simulink model "Radar410_Rx"  (R2018b)
settings: Solver=VariableStepAuto  StartTime=0.0  StopTime=10.0  RelTol=1e-3
PostLoadFcn:
  | if any(exist('dsrtsu_mdlpostloadfcn', 'file') ~= 0), dsrtsu_mdlpostloadfcn('Execute', bdroot); end
libraries: rtican x82
(part 24 of 24)

== system Radar410_Rx/Radar410_RX/Subsystem41/Subsystem40 ==
  In1 : Inport
  Bus Creator : BusCreator  Inputs=11  OutDataTypeStr=Bus: Radar_Status  NonVirtualBus=on
      settings: InheritFromInputs=off
  Bus Selector : BusSelector  OutputSignals=FRS_Msg_CheckSum,FRS_Msg_AliveCounter,FRS_Status_MisAlign,FRS_Status_HWErr,FRS_Status_BlkProg,FRS_Fail,FRS_MeasEnabled,FRS_Host_Yaw,FRS_HostSpeed,FRS_TimeStamp,FRS_Latency
  Data Type Conversion{,1..10} (11 alike) : DataTypeConversion  OutDataTypeStr=single
  Out1 : Outport  OutDataTypeStr=Bus: Radar_Status
  wires:
  Bus Selector/5 -> Data Type Conversion4/1  "<FRS_Status_BlkProg>"
  Bus Selector/8 -> Data Type Conversion7/1  "<FRS_Host_Yaw>"
  Bus Selector/1 -> Data Type Conversion/1  "<FRS_Msg_CheckSum>"
  Bus Selector/3 -> Data Type Conversion2/1  "<FRS_Status_MisAlign>"
  Bus Selector/2 -> Data Type Conversion1/1  "<FRS_Msg_AliveCounter>"
  Data Type Conversion5/1 -> Bus Creator/6
  Bus Selector/4 -> Data Type Conversion3/1  "<FRS_Status_HWErr>"
  Bus Selector/7 -> Data Type Conversion6/1  "<FRS_MeasEnabled>"
  Data Type Conversion9/1 -> Bus Creator/10
  Bus Selector/6 -> Data Type Conversion5/1  "<FRS_Fail>"
  Bus Selector/11 -> Data Type Conversion10/1  "<FRS_Latency>"
  Data Type Conversion6/1 -> Bus Creator/7
  Bus Selector/9 -> Data Type Conversion8/1  "<FRS_HostSpeed>"
  Bus Selector/10 -> Data Type Conversion9/1  "<FRS_TimeStamp>"
  Data Type Conversion10/1 -> Bus Creator/11
  In1/1 -> Bus Selector/1
  Bus Creator/1 -> Out1/1
  Data Type Conversion/1 -> Bus Creator/1
  Data Type Conversion2/1 -> Bus Creator/3
  Data Type Conversion1/1 -> Bus Creator/2
  Data Type Conversion4/1 -> Bus Creator/5
  Data Type Conversion3/1 -> Bus Creator/4
  Data Type Conversion7/1 -> Bus Creator/8
  Data Type Conversion8/1 -> Bus Creator/9

== system Radar410_Rx/Radar410_RX/Subsystem41/Subsystem5 ==
  In1 : Inport
  Bus Creator : BusCreator  Inputs=20  OutDataTypeStr=Bus: Obj_Data  NonVirtualBus=on
      settings: InheritFromInputs=off
  Bus Selector : BusSelector  OutputSignals=FRS_P1_05_Msg_CheckSum,FRS_P1_05_Msg_AliveCounter,FRS_P1_05_Obj_ExstProb,FRS_P1_05_Obj_XVelRel_Stdev,FRS_P1_05_Obj_XAccRel,FRS_P1_05_Obj_ObstacleProb,FRS_P1_05_Obj_MotionPattern,FRS_P1_05_Obj_YPos_Stdev,FRS_P1_05_Obj_ValidFlag,FRS_P1_05_Obj_XPos_Stdev,FRS_P1_05_Obj_UpdateFlag,FRS_P1_05_Obj_ID,FRS_P2_05_Msg_CheckSum,FRS_P2_05_Msg_AliveCounter,FRS_P2_05_Obj_MeasFlag,FRS_P2_05_Obj_YVelRel,FRS_P2_05_Obj_Type,FRS_P2_05_Obj_XPos,FRS_P2_05_Obj_YPos,FRS_P2_05_Obj_XVelRel
  Data Type Conversion{,1..19} (20 alike) : DataTypeConversion  OutDataTypeStr=single
  Out1 : Outport  OutDataTypeStr=Bus: Obj_Data
  wires:
  Data Type Conversion19/1 -> Bus Creator/20
  Data Type Conversion14/1 -> Bus Creator/15
  Data Type Conversion8/1 -> Bus Creator/9
  Data Type Conversion7/1 -> Bus Creator/8
  Data Type Conversion3/1 -> Bus Creator/4
  Data Type Conversion4/1 -> Bus Creator/5
  Data Type Conversion1/1 -> Bus Creator/2
  Data Type Conversion13/1 -> Bus Creator/14
  Data Type Conversion2/1 -> Bus Creator/3
  Data Type Conversion/1 -> Bus Creator/1
  Bus Creator/1 -> Out1/1
  In1/1 -> Bus Selector/1
  Bus Selector/20 -> Data Type Conversion19/1  "<FRS_P2_05_Obj_XVelRel>"
  Bus Selector/18 -> Data Type Conversion17/1  "<FRS_P2_05_Obj_XPos>"
  Bus Selector/19 -> Data Type Conversion18/1  "<FRS_P2_05_Obj_YPos>"
  Bus Selector/14 -> Data Type Conversion13/1  "<FRS_P2_05_Msg_AliveCounter>"
  Data Type Conversion10/1 -> Bus Creator/11
  Bus Selector/10 -> Data Type Conversion9/1  "<FRS_P1_05_Obj_XPos_Stdev>"
  Bus Selector/17 -> Data Type Conversion16/1  "<FRS_P2_05_Obj_Type>"
  Bus Selector/9 -> Data Type Conversion8/1  "<FRS_P1_05_Obj_ValidFlag>"
  Data Type Conversion16/1 -> Bus Creator/17
  Bus Selector/12 -> Data Type Conversion11/1  "<FRS_P1_05_Obj_ID>"
  Data Type Conversion6/1 -> Bus Creator/7
  Bus Selector/16 -> Data Type Conversion15/1  "<FRS_P2_05_Obj_YVelRel>"
  Data Type Conversion17/1 -> Bus Creator/18
  Bus Selector/11 -> Data Type Conversion10/1  "<FRS_P1_05_Obj_UpdateFlag>"
  Data Type Conversion18/1 -> Bus Creator/19
  Bus Selector/6 -> Data Type Conversion5/1  "<FRS_P1_05_Obj_ObstacleProb>"
  Data Type Conversion9/1 -> Bus Creator/10
  Bus Selector/7 -> Data Type Conversion6/1  "<FRS_P1_05_Obj_MotionPattern>"
  Bus Selector/4 -> Data Type Conversion3/1  "<FRS_P1_05_Obj_XVelRel_Stdev>"
  Data Type Conversion5/1 -> Bus Creator/6
  Data Type Conversion11/1 -> Bus Creator/12
  Bus Selector/2 -> Data Type Conversion1/1  "<FRS_P1_05_Msg_AliveCounter>"
  Bus Selector/13 -> Data Type Conversion12/1  "<FRS_P2_05_Msg_CheckSum>"
  Bus Selector/3 -> Data Type Conversion2/1  "<FRS_P1_05_Obj_ExstProb>"
  Bus Selector/15 -> Data Type Conversion14/1  "<FRS_P2_05_Obj_MeasFlag>"
  Bus Selector/1 -> Data Type Conversion/1  "<FRS_P1_05_Msg_CheckSum>"
  Data Type Conversion15/1 -> Bus Creator/16
  Bus Selector/8 -> Data Type Conversion7/1  "<FRS_P1_05_Obj_YPos_Stdev>"
  Bus Selector/5 -> Data Type Conversion4/1  "<FRS_P1_05_Obj_XAccRel>"
  Data Type Conversion12/1 -> Bus Creator/13

== system Radar410_Rx/Radar410_RX/Subsystem41/Subsystem6 ==
  In1 : Inport
  Bus Creator : BusCreator  Inputs=20  OutDataTypeStr=Bus: Obj_Data  NonVirtualBus=on
      settings: InheritFromInputs=off
  Bus Selector : BusSelector  OutputSignals=FRS_P1_06_Msg_CheckSum,FRS_P1_06_Msg_AliveCounter,FRS_P1_06_Obj_ExstProb,FRS_P1_06_Obj_XVelRel_Stdev,FRS_P1_06_Obj_XAccRel,FRS_P1_06_Obj_ObstacleProb,FRS_P1_06_Obj_MotionPattern,FRS_P1_06_Obj_YPos_Stdev,FRS_P1_06_Obj_ValidFlag,FRS_P1_06_Obj_XPos_Stdev,FRS_P1_06_Obj_UpdateFlag,FRS_P1_06_Obj_ID,FRS_P2_06_Msg_CheckSum,FRS_P2_06_Msg_AliveCounter,FRS_P2_06_Obj_MeasFlag,FRS_P2_06_Obj_YVelRel,FRS_P2_06_Obj_Type,FRS_P2_06_Obj_XPos,FRS_P2_06_Obj_YPos,FRS_P2_06_Obj_XVelRel
  Data Type Conversion{,1..19} (20 alike) : DataTypeConversion  OutDataTypeStr=single
  Out1 : Outport  OutDataTypeStr=Bus: Obj_Data
  wires:
  Data Type Conversion19/1 -> Bus Creator/20
  Data Type Conversion14/1 -> Bus Creator/15
  Data Type Conversion8/1 -> Bus Creator/9
  Data Type Conversion7/1 -> Bus Creator/8
  Data Type Conversion3/1 -> Bus Creator/4
  Data Type Conversion4/1 -> Bus Creator/5
  Data Type Conversion1/1 -> Bus Creator/2
  Data Type Conversion13/1 -> Bus Creator/14
  Data Type Conversion2/1 -> Bus Creator/3
  Data Type Conversion/1 -> Bus Creator/1
  Bus Creator/1 -> Out1/1
  In1/1 -> Bus Selector/1
  Bus Selector/20 -> Data Type Conversion19/1  "<FRS_P2_06_Obj_XVelRel>"
  Bus Selector/18 -> Data Type Conversion17/1  "<FRS_P2_06_Obj_XPos>"
  Bus Selector/19 -> Data Type Conversion18/1  "<FRS_P2_06_Obj_YPos>"
  Bus Selector/14 -> Data Type Conversion13/1  "<FRS_P2_06_Msg_AliveCounter>"
  Data Type Conversion10/1 -> Bus Creator/11
  Bus Selector/10 -> Data Type Conversion9/1  "<FRS_P1_06_Obj_XPos_Stdev>"
  Bus Selector/17 -> Data Type Conversion16/1  "<FRS_P2_06_Obj_Type>"
  Bus Selector/9 -> Data Type Conversion8/1  "<FRS_P1_06_Obj_ValidFlag>"
  Data Type Conversion16/1 -> Bus Creator/17
  Bus Selector/12 -> Data Type Conversion11/1  "<FRS_P1_06_Obj_ID>"
  Data Type Conversion6/1 -> Bus Creator/7
  Bus Selector/16 -> Data Type Conversion15/1  "<FRS_P2_06_Obj_YVelRel>"
  Data Type Conversion17/1 -> Bus Creator/18
  Bus Selector/11 -> Data Type Conversion10/1  "<FRS_P1_06_Obj_UpdateFlag>"
  Data Type Conversion18/1 -> Bus Creator/19
  Bus Selector/6 -> Data Type Conversion5/1  "<FRS_P1_06_Obj_ObstacleProb>"
  Data Type Conversion9/1 -> Bus Creator/10
  Bus Selector/7 -> Data Type Conversion6/1  "<FRS_P1_06_Obj_MotionPattern>"
  Bus Selector/4 -> Data Type Conversion3/1  "<FRS_P1_06_Obj_XVelRel_Stdev>"
  Data Type Conversion5/1 -> Bus Creator/6
  Data Type Conversion11/1 -> Bus Creator/12
  Bus Selector/2 -> Data Type Conversion1/1  "<FRS_P1_06_Msg_AliveCounter>"
  Bus Selector/13 -> Data Type Conversion12/1  "<FRS_P2_06_Msg_CheckSum>"
  Bus Selector/3 -> Data Type Conversion2/1  "<FRS_P1_06_Obj_ExstProb>"
  Bus Selector/15 -> Data Type Conversion14/1  "<FRS_P2_06_Obj_MeasFlag>"
  Bus Selector/1 -> Data Type Conversion/1  "<FRS_P1_06_Msg_CheckSum>"
  Data Type Conversion15/1 -> Bus Creator/16
  Bus Selector/8 -> Data Type Conversion7/1  "<FRS_P1_06_Obj_YPos_Stdev>"
  Bus Selector/5 -> Data Type Conversion4/1  "<FRS_P1_06_Obj_XAccRel>"
  Data Type Conversion12/1 -> Bus Creator/13

== system Radar410_Rx/Radar410_RX/Subsystem41/Subsystem7 ==
  In1 : Inport
  Bus Creator : BusCreator  Inputs=20  OutDataTypeStr=Bus: Obj_Data  NonVirtualBus=on
      settings: InheritFromInputs=off
  Bus Selector : BusSelector  OutputSignals=FRS_P1_07_Msg_CheckSum,FRS_P1_07_Msg_AliveCounter,FRS_P1_07_Obj_ExstProb,FRS_P1_07_Obj_XVelRel_Stdev,FRS_P1_07_Obj_XAccRel,FRS_P1_07_Obj_ObstacleProb,FRS_P1_07_Obj_MotionPattern,FRS_P1_07_Obj_YPos_Stdev,FRS_P1_07_Obj_ValidFlag,FRS_P1_07_Obj_XPos_Stdev,FRS_P1_07_Obj_UpdateFlag,FRS_P1_07_Obj_ID,FRS_P2_07_Msg_CheckSum,FRS_P2_07_Msg_AliveCounter,FRS_P2_07_Obj_MeasFlag,FRS_P2_07_Obj_YVelRel,FRS_P2_07_Obj_Type,FRS_P2_07_Obj_XPos,FRS_P2_07_Obj_YPos,FRS_P2_07_Obj_XVelRel
  Data Type Conversion{,1..19} (20 alike) : DataTypeConversion  OutDataTypeStr=single
  Out1 : Outport  OutDataTypeStr=Bus: Obj_Data
  wires:
  Data Type Conversion12/1 -> Bus Creator/13
  Bus Selector/5 -> Data Type Conversion4/1  "<FRS_P1_07_Obj_XAccRel>"
  Bus Selector/8 -> Data Type Conversion7/1  "<FRS_P1_07_Obj_YPos_Stdev>"
  Data Type Conversion15/1 -> Bus Creator/16
  Bus Selector/1 -> Data Type Conversion/1  "<FRS_P1_07_Msg_CheckSum>"
  Bus Selector/15 -> Data Type Conversion14/1  "<FRS_P2_07_Obj_MeasFlag>"
  Bus Selector/3 -> Data Type Conversion2/1  "<FRS_P1_07_Obj_ExstProb>"
  Bus Selector/13 -> Data Type Conversion12/1  "<FRS_P2_07_Msg_CheckSum>"
  Bus Selector/2 -> Data Type Conversion1/1  "<FRS_P1_07_Msg_AliveCounter>"
  Data Type Conversion11/1 -> Bus Creator/12
  Data Type Conversion5/1 -> Bus Creator/6
  Bus Selector/4 -> Data Type Conversion3/1  "<FRS_P1_07_Obj_XVelRel_Stdev>"
  Bus Selector/7 -> Data Type Conversion6/1  "<FRS_P1_07_Obj_MotionPattern>"
  Data Type Conversion9/1 -> Bus Creator/10
  Bus Selector/6 -> Data Type Conversion5/1  "<FRS_P1_07_Obj_ObstacleProb>"
  Data Type Conversion18/1 -> Bus Creator/19
  Bus Selector/11 -> Data Type Conversion10/1  "<FRS_P1_07_Obj_UpdateFlag>"
  Data Type Conversion17/1 -> Bus Creator/18
  Bus Selector/16 -> Data Type Conversion15/1  "<FRS_P2_07_Obj_YVelRel>"
  Data Type Conversion6/1 -> Bus Creator/7
  Bus Selector/12 -> Data Type Conversion11/1  "<FRS_P1_07_Obj_ID>"
  Data Type Conversion16/1 -> Bus Creator/17
  Bus Selector/9 -> Data Type Conversion8/1  "<FRS_P1_07_Obj_ValidFlag>"
  Bus Selector/17 -> Data Type Conversion16/1  "<FRS_P2_07_Obj_Type>"
  Bus Selector/10 -> Data Type Conversion9/1  "<FRS_P1_07_Obj_XPos_Stdev>"
  Data Type Conversion10/1 -> Bus Creator/11
  Bus Selector/14 -> Data Type Conversion13/1  "<FRS_P2_07_Msg_AliveCounter>"
  Bus Selector/19 -> Data Type Conversion18/1  "<FRS_P2_07_Obj_YPos>"
  Bus Selector/18 -> Data Type Conversion17/1  "<FRS_P2_07_Obj_XPos>"
  Bus Selector/20 -> Data Type Conversion19/1  "<FRS_P2_07_Obj_XVelRel>"
  In1/1 -> Bus Selector/1
  Bus Creator/1 -> Out1/1
  Data Type Conversion/1 -> Bus Creator/1
  Data Type Conversion2/1 -> Bus Creator/3
  Data Type Conversion13/1 -> Bus Creator/14
  Data Type Conversion1/1 -> Bus Creator/2
  Data Type Conversion4/1 -> Bus Creator/5
  Data Type Conversion3/1 -> Bus Creator/4
  Data Type Conversion7/1 -> Bus Creator/8
  Data Type Conversion8/1 -> Bus Creator/9
  Data Type Conversion14/1 -> Bus Creator/15
  Data Type Conversion19/1 -> Bus Creator/20

== system Radar410_Rx/Radar410_RX/Subsystem41/Subsystem8 ==
  In1 : Inport
  Bus Creator : BusCreator  Inputs=20  OutDataTypeStr=Bus: Obj_Data  NonVirtualBus=on
      settings: InheritFromInputs=off
  Bus Selector : BusSelector  OutputSignals=FRS_P1_08_Msg_CheckSum,FRS_P1_08_Msg_AliveCounter,FRS_P1_08_Obj_ExstProb,FRS_P1_08_Obj_XVelRel_Stdev,FRS_P1_08_Obj_XAccRel,FRS_P1_08_Obj_ObstacleProb,FRS_P1_08_Obj_MotionPattern,FRS_P1_08_Obj_YPos_Stdev,FRS_P1_08_Obj_ValidFlag,FRS_P1_08_Obj_XPos_Stdev,FRS_P1_08_Obj_UpdateFlag,FRS_P1_08_Obj_ID,FRS_P2_08_Msg_CheckSum,FRS_P2_08_Msg_AliveCounter,FRS_P2_08_Obj_MeasFlag,FRS_P2_08_Obj_YVelRel,FRS_P2_08_Obj_Type,FRS_P2_08_Obj_XPos,FRS_P2_08_Obj_YPos,FRS_P2_08_Obj_XVelRel
  Data Type Conversion{,1..19} (20 alike) : DataTypeConversion  OutDataTypeStr=single
  Out1 : Outport  OutDataTypeStr=Bus: Obj_Data
  wires:
  Data Type Conversion12/1 -> Bus Creator/13
  Bus Selector/5 -> Data Type Conversion4/1  "<FRS_P1_08_Obj_XAccRel>"
  Bus Selector/8 -> Data Type Conversion7/1  "<FRS_P1_08_Obj_YPos_Stdev>"
  Data Type Conversion15/1 -> Bus Creator/16
  Bus Selector/1 -> Data Type Conversion/1  "<FRS_P1_08_Msg_CheckSum>"
  Bus Selector/15 -> Data Type Conversion14/1  "<FRS_P2_08_Obj_MeasFlag>"
  Bus Selector/3 -> Data Type Conversion2/1  "<FRS_P1_08_Obj_ExstProb>"
  Bus Selector/13 -> Data Type Conversion12/1  "<FRS_P2_08_Msg_CheckSum>"
  Bus Selector/2 -> Data Type Conversion1/1  "<FRS_P1_08_Msg_AliveCounter>"
  Data Type Conversion11/1 -> Bus Creator/12
  Data Type Conversion5/1 -> Bus Creator/6
  Bus Selector/4 -> Data Type Conversion3/1  "<FRS_P1_08_Obj_XVelRel_Stdev>"
  Bus Selector/7 -> Data Type Conversion6/1  "<FRS_P1_08_Obj_MotionPattern>"
  Data Type Conversion9/1 -> Bus Creator/10
  Bus Selector/6 -> Data Type Conversion5/1  "<FRS_P1_08_Obj_ObstacleProb>"
  Data Type Conversion18/1 -> Bus Creator/19
  Bus Selector/11 -> Data Type Conversion10/1  "<FRS_P1_08_Obj_UpdateFlag>"
  Data Type Conversion17/1 -> Bus Creator/18
  Bus Selector/16 -> Data Type Conversion15/1  "<FRS_P2_08_Obj_YVelRel>"
  Data Type Conversion6/1 -> Bus Creator/7
  Bus Selector/12 -> Data Type Conversion11/1  "<FRS_P1_08_Obj_ID>"
  Data Type Conversion16/1 -> Bus Creator/17
  Bus Selector/9 -> Data Type Conversion8/1  "<FRS_P1_08_Obj_ValidFlag>"
  Bus Selector/17 -> Data Type Conversion16/1  "<FRS_P2_08_Obj_Type>"
  Bus Selector/10 -> Data Type Conversion9/1  "<FRS_P1_08_Obj_XPos_Stdev>"
  Data Type Conversion10/1 -> Bus Creator/11
  Bus Selector/14 -> Data Type Conversion13/1  "<FRS_P2_08_Msg_AliveCounter>"
  Bus Selector/19 -> Data Type Conversion18/1  "<FRS_P2_08_Obj_YPos>"
  Bus Selector/18 -> Data Type Conversion17/1  "<FRS_P2_08_Obj_XPos>"
  Bus Selector/20 -> Data Type Conversion19/1  "<FRS_P2_08_Obj_XVelRel>"
  In1/1 -> Bus Selector/1
  Bus Creator/1 -> Out1/1
  Data Type Conversion/1 -> Bus Creator/1
  Data Type Conversion2/1 -> Bus Creator/3
  Data Type Conversion13/1 -> Bus Creator/14
  Data Type Conversion1/1 -> Bus Creator/2
  Data Type Conversion4/1 -> Bus Creator/5
  Data Type Conversion3/1 -> Bus Creator/4
  Data Type Conversion7/1 -> Bus Creator/8
  Data Type Conversion8/1 -> Bus Creator/9
  Data Type Conversion14/1 -> Bus Creator/15
  Data Type Conversion19/1 -> Bus Creator/20

== system Radar410_Rx/Radar410_RX/Subsystem41/Subsystem9 ==
  In1 : Inport
  Bus Creator : BusCreator  Inputs=20  OutDataTypeStr=Bus: Obj_Data  NonVirtualBus=on
      settings: InheritFromInputs=off
  Bus Selector : BusSelector  OutputSignals=FRS_P1_09_Msg_CheckSum,FRS_P1_09_Msg_AliveCounter,FRS_P1_09_Obj_ExstProb,FRS_P1_09_Obj_XVelRel_Stdev,FRS_P1_09_Obj_XAccRel,FRS_P1_09_Obj_ObstacleProb,FRS_P1_09_Obj_MotionPattern,FRS_P1_09_Obj_YPos_Stdev,FRS_P1_09_Obj_ValidFlag,FRS_P1_09_Obj_XPos_Stdev,FRS_P1_09_Obj_UpdateFlag,FRS_P1_09_Obj_ID,FRS_P2_09_Msg_CheckSum,FRS_P2_09_Msg_AliveCounter,FRS_P2_09_Obj_MeasFlag,FRS_P2_09_Obj_YVelRel,FRS_P2_09_Obj_Type,FRS_P2_09_Obj_XPos,FRS_P2_09_Obj_YPos,FRS_P2_09_Obj_XVelRel
  Data Type Conversion{,1..19} (20 alike) : DataTypeConversion  OutDataTypeStr=single
  Out1 : Outport  OutDataTypeStr=Bus: Obj_Data
  wires:
  Data Type Conversion19/1 -> Bus Creator/20
  Data Type Conversion14/1 -> Bus Creator/15
  Data Type Conversion8/1 -> Bus Creator/9
  Data Type Conversion7/1 -> Bus Creator/8
  Data Type Conversion3/1 -> Bus Creator/4
  Data Type Conversion4/1 -> Bus Creator/5
  Data Type Conversion1/1 -> Bus Creator/2
  Data Type Conversion13/1 -> Bus Creator/14
  Data Type Conversion2/1 -> Bus Creator/3
  Data Type Conversion/1 -> Bus Creator/1
  Bus Creator/1 -> Out1/1
  In1/1 -> Bus Selector/1
  Bus Selector/20 -> Data Type Conversion19/1  "<FRS_P2_09_Obj_XVelRel>"
  Bus Selector/18 -> Data Type Conversion17/1  "<FRS_P2_09_Obj_XPos>"
  Bus Selector/19 -> Data Type Conversion18/1  "<FRS_P2_09_Obj_YPos>"
  Bus Selector/14 -> Data Type Conversion13/1  "<FRS_P2_09_Msg_AliveCounter>"
  Data Type Conversion10/1 -> Bus Creator/11
  Bus Selector/10 -> Data Type Conversion9/1  "<FRS_P1_09_Obj_XPos_Stdev>"
  Bus Selector/17 -> Data Type Conversion16/1  "<FRS_P2_09_Obj_Type>"
  Bus Selector/9 -> Data Type Conversion8/1  "<FRS_P1_09_Obj_ValidFlag>"
  Data Type Conversion16/1 -> Bus Creator/17
  Bus Selector/12 -> Data Type Conversion11/1  "<FRS_P1_09_Obj_ID>"
  Data Type Conversion6/1 -> Bus Creator/7
  Bus Selector/16 -> Data Type Conversion15/1  "<FRS_P2_09_Obj_YVelRel>"
  Data Type Conversion17/1 -> Bus Creator/18
  Bus Selector/11 -> Data Type Conversion10/1  "<FRS_P1_09_Obj_UpdateFlag>"
  Data Type Conversion18/1 -> Bus Creator/19
  Bus Selector/6 -> Data Type Conversion5/1  "<FRS_P1_09_Obj_ObstacleProb>"
  Data Type Conversion9/1 -> Bus Creator/10
  Bus Selector/7 -> Data Type Conversion6/1  "<FRS_P1_09_Obj_MotionPattern>"
  Bus Selector/4 -> Data Type Conversion3/1  "<FRS_P1_09_Obj_XVelRel_Stdev>"
  Data Type Conversion5/1 -> Bus Creator/6
  Data Type Conversion11/1 -> Bus Creator/12
  Bus Selector/2 -> Data Type Conversion1/1  "<FRS_P1_09_Msg_AliveCounter>"
  Bus Selector/13 -> Data Type Conversion12/1  "<FRS_P2_09_Msg_CheckSum>"
  Bus Selector/3 -> Data Type Conversion2/1  "<FRS_P1_09_Obj_ExstProb>"
  Bus Selector/15 -> Data Type Conversion14/1  "<FRS_P2_09_Obj_MeasFlag>"
  Bus Selector/1 -> Data Type Conversion/1  "<FRS_P1_09_Msg_CheckSum>"
  Data Type Conversion15/1 -> Bus Creator/16
  Bus Selector/8 -> Data Type Conversion7/1  "<FRS_P1_09_Obj_YPos_Stdev>"
  Bus Selector/5 -> Data Type Conversion4/1  "<FRS_P1_09_Obj_XAccRel>"
  Data Type Conversion12/1 -> Bus Creator/13
